simulink model "PMSM_18bMRASV20190225"  (R2020a)
settings: Solver=ode3  StartTime=0.0  StopTime=50  FixedStep=Ts  MaxStep=2e-5  MinStep=1e-5  RelTol=2e-3
InitFcn:
  | Ld=8.9e-3;
  | Lq=12.7e-3;
  | L=(Ld+Lq)/2;
  | poles=3;
  | R=0.85;
  | flux=0.1216;
  | Ts=1e-5;
model workspace (MAT data in the model file):
  Tl2 = [0 -0.0065 -0.013 -0.0195 -0.026 -0.0325 -0.039 -0.0455 -0.052 -0.0585 -0.065 -0.0715 ... (360 elements, 1x360)]
libraries: powerlib x19, powerlib_extras x16, simulink x8
settings Model: SimulationMode=accelerator  Creator=Paladin611  LastModifiedBy=Administrator
settings SolverCC: InitialStep=1e-5  MaxConsecutiveZCs=2000  ShapePreserveControl=EnableAll  AutoInsertRateTranBlk=on  InsertRTBMode=Always
settings DataIOCC: SaveFormat=Array  ReturnWorkspaceOutputs=off
settings OptimizationCC: DefaultParameterBehavior=Inlined  EnhancedBackFolding=on  PassReuseOutputArgsAs=Individual arguments  ExpressionDepthLimit=2147483647  ZeroExternalMemoryAtStartup=off  ZeroInternalMemoryAtStartup=off  InitFltsAndDblsToZero=on  EfficientMapNaN2IntZero=off  OptimizeBlockOrder=speed  DifferentSizesBufferReuse=on  OptimizationCustomize=off  EfficientTunableParamExpr=on
settings DebuggingCC: SaveWithParameterizedLinksMsg=none  UnderspecifiedInitializationDetection=Classic  MergeDetectMultiDrivingBlocksExec=none  SignalResolutionControl=TryResolveAllWithWarning  SolverPrmCheckMsg=warning  MultiTaskCondExecSysMsg=none  ParameterTunabilityLossMsg=error  FcnCallInpInsideContextMsg=warning  StateNameClashWarn=warning  SFUnexpectedBacktrackingDiag=warning  SFNoUnconditionalDefaultTransitionDiag=warning  SFExecutionAtInitializationDiag=none  ArithmeticOperatorsInVariantConditions=warning
settings HardwareCC: ProdBitPerPointer=32  ProdBitPerSizeT=32  ProdBitPerPtrDiffT=32  ProdLargestAtomicFloat=None  ProdIntDivRoundTo=Undefined  ProdEndianess=Unspecified  ProdWordSize=32  ProdHWDeviceType=32-bit Generic  TargetBitPerPointer=64  TargetBitPerSizeT=64  TargetBitPerPtrDiffT=64  TargetLongLongMode=on  TargetIntDivRoundTo=Zero  TargetEndianess=LittleEndian  TargetWordSize=64  TargetHWDeviceType=MATLAB Host  ProdEqTarget=off
settings ModelReferenceCC: PropagateSignalLabelsOutOfModel=off
settings SFSimCC: SimUseLocalCustomCode=off  MATLABDynamicMemAlloc=off  CustomCodeUndefinedFunction=UseInterfaceOnly
settings RTWCC: SystemTargetFile=ert.tlc  TemplateMakefile=ert_default_tmf  GenerateReport=on  RTWUseLocalCustomCode=off  IncludeHyperlinkInReport=on  LaunchReport=on  GenerateTraceInfo=on  GenerateTraceReport=on  GenerateTraceReportSl=on  GenerateTraceReportSf=on  GenerateTraceReportEml=on
settings CodeAppCC: ForceParamTrailComments=on  IgnoreCustomStorageClasses=off  MaxIdLength=128  OperatorAnnotations=on  SimulinkDataObjDesc=on  SFDataObjDesc=on  InsertBlockDesc=on
settings ERTTargetCC: GenerateSampleERTMain=on  InlinedParameterPlacement=NonHierarchical  ERTCustomFileTemplate=example_file_process.tlc
settings ConfigComp: CovMetricSettings=dw  CovHtmlReporting=on  CovSaveCumulativeToWorkspaceVar=on  CovSaveSingleToWorkspaceVar=on  CovExternalEMLEnable=off  CovSFcnEnable=off
settings SimscapeCC: SimscapeNormalizeSystem=off

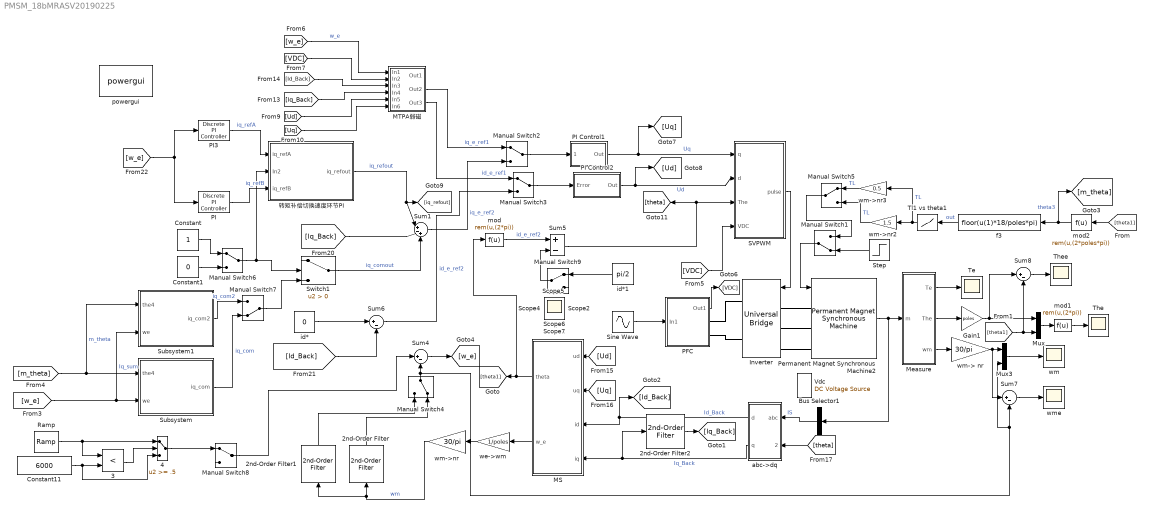
== system PMSM_18bMRASV20190225 ==
  "  3" : RelationalOperator  Operator=<  OutDataTypeStr=boolean  RndMeth=Nearest
  " Tl1 vs theta1" : Lookup  InputValues=0:359  Table=Tl2
  2nd-Order Filter : powerlib_extras/Control  Blocks/2nd-Order Filter  FilterType=Lowpass  Fo=30  Zeta=0.707  Initialize=off  Vac_Init=[1 45 60]  Vdc_Init=-0.5  PlotResponse=off  param1=[1 500 1]
      settings: SourceProductBaseCode=PS
  2nd-Order Filter1 : powerlib_extras/Control  Blocks/2nd-Order Filter  FilterType=Lowpass  Fo=800  Zeta=0.707  Initialize=off  Vac_Init=[1 45 60]  Vdc_Init=-0.5  PlotResponse=off  param1=[1 500 1]
      settings: SourceProductBaseCode=PS
  2nd-Order Filter2 : powerlib_extras/Control  Blocks/2nd-Order Filter  FilterType=Lowpass  Fo=800  Zeta=0.707  Initialize=off  Vac_Init=[1 45 60]  Vdc_Init=-0.5  PlotResponse=off  param1=[1 500 1]
      settings: SourceProductBaseCode=PS
  4 : Switch  Threshold=.5
  Bus Selector1 : BusSelector  OutputSignals=Stator current is_a (A),Stator current is_b (A),Stator current is_c (A)  OutputAsBus=on
  Constant : Constant
  Constant1 : Constant  Value=0
  Constant11 : Constant  Value=6000
  Gain1 : Gain  Gain=poles
  Inverter : powerlib/Power Electronics/Universal Bridge  Arms=3  SnubberResistance=1e5  SnubberCapacitance=inf  Device=IGBT / Diodes  Ron=1e-3  Lon=0  ForwardVoltages="[  0  0  ]"  ForwardVoltage=0  GTOparameters=[ 10e-6 , 20e-6 ]  IGBTparameters=[ 1e-6 , 2e-6 ]  Measurements=None  Measurements_2=None  converterType=Rectifier
  MS : Subsystem
  MTPA弱磁 : Subsystem
  Manual Switch1 : ManualSwitch  CurrentSetting=0
  Manual Switch{2..3,5..6,8..9} (6 alike) : ManualSwitch
  Manual Switch4 : ManualSwitch  CurrentSetting=0
  Manual Switch7 : ManualSwitch  CurrentSetting=0
  Measure : Subsystem
  Mux : Mux  Inputs=2
  Mux3 : Mux  Inputs=2
  PFC : Subsystem
  PI : powerlib_extras/Discrete  Control Blocks/Discrete PI Controller  Kp=0.002  Ki=0.0002  Par_Limits=[200 -200]  Init=0  Ts=Ts
  PI Control1 : Subsystem  mask(PI Control){Kp=Lq*2000, Ki=R*2000, Kc=3, UpperLimit=400, LowerLimit=-400}
      mask prompts: Kp "PI_Kp:"; Ki "PI_Ki:"; Kc "PI_Kc:"; UpperLimit "MAX:"; LowerLimit "MIN:"
      mask help:
      | PI Control
      |
      | CopyRight:maxthonzwq 2012/03/22
  PI Control2 : Subsystem  mask(PI Control){Kp=Ld*2000, Ki=R*2000, Kc=3, UpperLimit=400, LowerLimit=-400}
      mask prompts: Kp "PI_Kp:"; Ki "PI_Ki:"; Kc "PI_Kc:"; UpperLimit "MAX:"; LowerLimit "MIN:"
      mask help:
      | PI Control
      |
      | CopyRight:maxthonzwq 2012/03/22
  PI3 : powerlib_extras/Discrete  Control Blocks/Discrete PI Controller  Kp=0.03  Ki=0.002  Par_Limits=[200 -200]  Init=0  Ts=Ts
  Permanent Magnet Synchronous Machine2 : powerlib/Machines/Permanent Magnet Synchronous Machine  NbPhases=3  FluxDistribution=Sinusoidal  RotorType=Salient-pole  MechanicalLoad=Torque Tm  PresetModel=No  ShowDetailedParameters=on  MeasurementBus=off  Resistance=R  Inductance=8.5e-3  dqInductances=[Ld Lq]  La=0.00085  MachineConstant=Flux linkage established by magnets (V.s)  Flux=0.175  VoltageCst=126.966  TorqueCst=1.05  Flat=120  Mechanical=[3.4e-4,0,poles,0]  PolePairs=4  InitialConditions=[0,0, 0,0]  InitialConditions5ph=[0 0 0 0 0 0]  RefAngle=Aligned with phase A axis (original Park)  IterativeDiscreteModel=Trapezoidal non iterative  TsBlock=-1  TsPowergui=0
  Ramp : simulink/Sources/Ramp  slope=1000  start=0  InitialOutput=1
  SVPWM : Subsystem
  Sine Wave : Sin  Frequency=50*2*pi  SampleTime=0
  Step : Step  Time=0  Before=0.3  SampleTime=0
  Subsystem : Subsystem
  Subsystem1 : Subsystem
  Sum1 : Sum  Inputs=|+-+
  Sum{4,6..8} (4 alike) : Sum  Inputs=|+-
  Sum5 : Sum  Inputs=+-
  Switch1 : Switch  Criteria=u2 > Threshold
  Te : Scope
  The : Scope
  Thee : Scope
  Vdc : powerlib/Electrical Sources/DC Voltage Source  Amplitude=311  Measurements=None
  abc->dq : Subsystem
  f3 : Fcn  Expr=floor(u(1)*18/poles*pi)  SampleTime=0.0001
  id* : Constant  Value=0
  id*1 : Constant  Value=pi/2
  mod : Fcn  Expr=rem(u,(2*pi))
  mod1 : Fcn  Expr=rem(u,(2*pi))
  mod2 : Fcn  Expr=rem(u,(2*poles*pi))
  powergui : powerlib/powergui  Priority=1  SimulationMode=Discrete  SampleTime=Ts  frequency=60  Iterations=50  frequencyindice=0  Pbase=100e6  ErrMax=1e-4  UnitsV=kV  UnitsW=MW  buscounter=0  FunctionMessages=off  echomessages=off  EnableUseOfTLC=off  CurrentSourceSwitches=on  DisableSnubberDevices=off  DisableRonSwitches=off  DisableVfSwitches=off  DisplayEquations=off  AutomaticDiscreteSolvers=off  SolverType=Tustin  Interpol=off  ExternalGateDelay=off  methode=off  Ts=0  x0status=blocks  SPID=off  SwTol=0  HookPort=off  NonlinearTolerance=1e-4  nMaxIteration=100  ContinueOnMaxIteration=off  RestoreLinks=warning  ResistiveCurrentMeasurement=off  Frange=[0:2:500]  Ylog=off  Xlog=on  ShowGrid=off  save=off  variable=ZData  structure=0  ZoomFFT=off  StartTime=0.0  cycles=1  DisplayStyle=1  fundamental=60  FreqAxis=off  MaxFrequency=1000  frequencyindicesteady=1  RmsSteady=1  display=off
  we->wm : Gain  Gain=1/poles
  wm : Scope
  wm-> nr : Gain  Gain=30/pi
  wm->nr : Gain  Gain=30/pi
  wm->nr2 : Gain  Gain=1.5
  wm->nr3 : Gain  Gain=0.5
  wme : Scope
  转矩补偿切换速度环节PI : Subsystem
  Scope{,1..2,4..7} (7 alike) : Scope
  wires:
  Permanent Magnet Synchronous Machine2/1 -> Measure/1(m), Bus Selector1/1
  id*/1 -> Sum6/1
  SVPWM/1(pulse) -> Inverter/1
  abc->dq/2(q) -> 2nd-Order Filter2/1, MS/4(iq)  "Iq_Back"
  MS/2(w_e) -> we->wm/1
  we->wm/1 -> wm->nr/1
  PI Control1/1(Out) -> SVPWM/1(q), [Uq]  "Uq"
  PI Control2/1(Out) -> [Ud], SVPWM/2(d)  "Ud"
  Measure/1(Te) -> Te/1
  Measure/2(The) -> Gain1/1
  Bus Selector1/1 -> abc->dq/1(abc)  "IS"
  Measure/3(wm) -> wm-> nr/1
  f3/1 -> " Tl1 vs theta1"/1  "out"
  [theta1] -> mod2/1
  Switch1/1 -> Sum1/3  "iq_comout"
  mod2/1 -> [m_theta], f3/1  "theta3"
  Step/1 -> Manual Switch1/2
  " Tl1 vs theta1"/1 -> wm->nr2/1, wm->nr3/1  "TL"
  PI3/1 -> 转矩补偿切换速度环节PI/1(iq_refA)  "iq_refA"
  Manual Switch6/1 -> 转矩补偿切换速度环节PI/2(In2), Switch1/2
  PI/1 -> 转矩补偿切换速度环节PI/3(iq_refB)  "iq_refB"
  转矩补偿切换速度环节PI/1(iq_refout) -> [iq_refout], Sum1/1  "iq_refout"
  [VDC] -> SVPWM/4(VDC)
  [Ud] -> MS/1(ud)
  [Uq] -> MS/2(uq)
  [theta] -> abc->dq/2(theta)
  [Id_Back] -> Sum6/2
  [Iq_Back] -> Sum1/2
  [w_e] -> PI/1, PI3/1
  Sine Wave/1 -> PFC/1(In1)
  Sum1/1 -> Manual Switch2/2  "iq_e_ref2"
  Manual Switch3/1 -> PI Control2/1(Error)
  Sum6/1 -> Manual Switch3/2  "id_e_ref2"
  [VDC] -> MTPA弱磁/2(In2)
  MTPA弱磁/2(Out2) -> Manual Switch2/1  "iq_e_ref1"
  MTPA弱磁/3(Out3) -> Manual Switch3/1  "id_e_ref1"
  [Id_Back] -> MTPA弱磁/3(In3)
  [Iq_Back] -> MTPA弱磁/4(In4)
  [Ud] -> MTPA弱磁/5(In5)
  [Uq] -> MTPA弱磁/6(In6)
  PFC/1(Out1) -> [VDC]
  abc->dq/1(d) -> MS/3(id), [Id_Back]  "Id_Back"
  Sum4/1 -> [w_e]
  [w_e] -> MTPA弱磁/1(In1)  "w_e"
  2nd-Order Filter/1 -> Manual Switch4/2
  wm->nr/1 -> 2nd-Order Filter1/1, 2nd-Order Filter/1  "wm"
  [m_theta] -> Subsystem/1(the4), Subsystem1/1(the4)  "m_theta"
  [w_e] -> Subsystem/2(we), Subsystem1/2(we)  "Iq_sum"
  Manual Switch1/1 -> Permanent Magnet Synchronous Machine2/1
  Manual Switch5/1 -> Manual Switch1/1
  wm->nr2/1 -> Manual Switch5/2  "TL"
  wm->nr3/1 -> Manual Switch5/1  "TL"
  Constant/1 -> Manual Switch6/1
  Constant1/1 -> Manual Switch6/2
  Subsystem1/1(iq_com2) -> Manual Switch7/1  "iq_com2"
  Subsystem/1(iq_com) -> Manual Switch7/2  "iq_com"
  Manual Switch7/1 -> Switch1/3
  2nd-Order Filter1/1 -> Manual Switch4/1
  2nd-Order Filter2/1 -> [Iq_Back]
  4/1 -> Manual Switch8/1
  Ramp/1 -> "  3"/1, 4/1
  Constant11/1 -> "  3"/2, 4/3
  "  3"/1 -> 4/2
  Manual Switch8/1 -> Sum4/1
  Manual Switch2/1 -> PI Control1/1(Error)
  Mux3/1 -> wm/1
  Sum7/1 -> wme/1
  Manual Switch4/1 -> Mux3/2, Sum7/2, Sum4/2
  Sum8/1 -> Thee/1
  wm-> nr/1 -> Sum7/1, Mux3/1
  mod1/1 -> The/1
  Mux/1 -> mod1/1
  MS/1(theta) -> mod/1, [theta1]
  Gain1/1 -> Mux/1, Sum8/1
  mod/1 -> Sum5/1  "id_e_ref2"
  Sum5/1 -> SVPWM/3(The), [theta]
  Manual Switch9/1 -> Sum5/2
  id*1/1 -> Manual Switch9/1
  [theta1] -> Sum8/2, Mux/2
  connections:
  Permanent Magnet Synchronous Machine2/LConn1 -- Inverter/LConn1
  Permanent Magnet Synchronous Machine2/LConn2 -- Inverter/LConn2
  Permanent Magnet Synchronous Machine2/LConn3 -- Inverter/LConn3
  Inverter/RConn1 -- PFC/RConn1
  Inverter/RConn2 -- PFC/RConn2

== system PMSM_18bMRASV20190225/MS ==
  ud : Inport
  uq : Inport  Port=2
  id : Inport  Port=3
  iq : Inport  Port=4
  Integrator : Integrator
  MRAS : Subsystem
  Manual Switch1 : ManualSwitch  CurrentSetting=0
  we : Subsystem
  we1 : Subsystem
  theta : Outport  VectorParamsAs1DForOutWhenUnconnected=off
  w_e : Outport  Port=2  VectorParamsAs1DForOutWhenUnconnected=off
  wires:
  ud/1 -> MRAS/1(ud)
  iq/1 -> we/2(iq), we1/2(iq)
  uq/1 -> MRAS/2(uq)
  Integrator/1 -> theta/1
  MRAS/2(i_q) -> we/4(i_q), we1/4(i_q)
  MRAS/1(i_d) -> we/3(i_d), we1/3(i_d)
  id/1 -> we/1(id), we1/1(id)
  Manual Switch1/1 -> MRAS/3(we), w_e/1, Integrator/1
  we/1(w_e) -> Manual Switch1/2
  we1/1(w_e) -> Manual Switch1/1

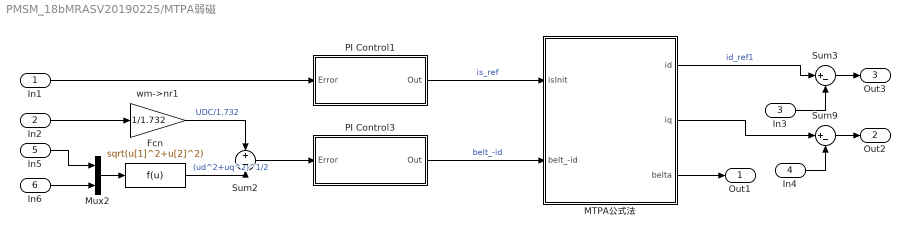
== system PMSM_18bMRASV20190225/MTPA弱磁 ==
  In1 : Inport
  In2 : Inport  Port=2
  In3 : Inport  Port=3
  In4 : Inport  Port=4
  In5 : Inport  Port=5
  In6 : Inport  Port=6
  Fcn : Fcn  Expr=sqrt(u[1]^2+u[2]^2)
  MTPA公式法 : Subsystem
  Mux2 : Mux  Inputs=2
  PI Control1 : Subsystem  mask(PI Control){Kp=0.05, Ki=0.004, Kc=3, UpperLimit=200, LowerLimit=-200}
      mask prompts: Kp "PI_Kp:"; Ki "PI_Ki:"; Kc "PI_Kc:"; UpperLimit "MAX:"; LowerLimit "MIN:"
      mask help:
      | PI Control
      |
      | CopyRight:maxthonzwq 2012/03/22
  PI Control3 : Subsystem  mask(PI Control){Kp=0.05, Ki=0.002, Kc=3, UpperLimit=200, LowerLimit=-200}
      mask prompts: Kp "PI_Kp:"; Ki "PI_Ki:"; Kc "PI_Kc:"; UpperLimit "MAX:"; LowerLimit "MIN:"
      mask help:
      | PI Control
      |
      | CopyRight:maxthonzwq 2012/03/22
  Sum2 : Sum  Inputs=+-
  Sum3 : Sum  Inputs=|+-
  Sum9 : Sum  Inputs=|+-
  wm->nr1 : Gain  Gain=1/1.732
  Out1 : Outport  VectorParamsAs1DForOutWhenUnconnected=off
  Out2 : Outport  Port=2  VectorParamsAs1DForOutWhenUnconnected=off
  Out3 : Outport  Port=3  VectorParamsAs1DForOutWhenUnconnected=off
  wires:
  wm->nr1/1 -> Sum2/1  "UDC/1.732"
  Fcn/1 -> Sum2/2  "(ud^2+uq^2)^1/2"
  PI Control3/1(Out) -> MTPA公式法/2(belt_-id)  "belt_-id"
  Sum2/1 -> PI Control3/1(Error)
  MTPA公式法/3(belta) -> Out1/1
  Sum3/1 -> Out3/1
  MTPA公式法/2(iq) -> Sum9/1
  Mux2/1 -> Fcn/1
  MTPA公式法/1(id) -> Sum3/1  "id_ref1"
  In3/1 -> Sum3/2
  Sum9/1 -> Out2/1
  In5/1 -> Mux2/1
  In2/1 -> wm->nr1/1
  In4/1 -> Sum9/2
  In1/1 -> PI Control1/1(Error)
  In6/1 -> Mux2/2
  PI Control1/1(Out) -> MTPA公式法/1(isInit)  "is_ref"

== system PMSM_18bMRASV20190225/Measure ==
  m : Inport
  Bus Selector : BusSelector  OutputSignals=Electromagnetic torque Te (N*m),Rotor angle thetam (rad),Rotor speed wm (rad/s)
  Te : Outport  VectorParamsAs1DForOutWhenUnconnected=off
  The : Outport  Port=2  VectorParamsAs1DForOutWhenUnconnected=off
  wm : Outport  Port=3  VectorParamsAs1DForOutWhenUnconnected=off
  wires:
  Bus Selector/1 -> Te/1  "<Electromagnetic torque Te (N*m)>"
  Bus Selector/3 -> wm/1  "<Rotor speed wm (rad/s)>"
  Bus Selector/2 -> The/1  "<Rotor angle thetam (rad)>"
  m/1 -> Bus Selector/1

== system PMSM_18bMRASV20190225/PFC ==
  In1 : Inport
  2nd-Order Filter : powerlib_extras/Control  Blocks/2nd-Order Filter  FilterType=Lowpass  Fo=20  Zeta=0.707  Initialize=off  Vac_Init=[1 45 60]  Vdc_Init=-0.5  PlotResponse=off  param1=[1 500 1]
      settings: SourceProductBaseCode=PS
  Constant : Constant  Value=350
  PFC : Subsystem
  Sum11 : Sum  Inputs=|-+
  Voltage Measurement1 : powerlib/Measurements/Voltage Measurement  PhasorSimulation=off  OutputType=Complex  PSBequivalent=0
  Conn1 : PMIOPort  Side=Right
  Conn2 : PMIOPort  Port=2  Side=Right
  Out1 : Outport  VectorParamsAs1DForOutWhenUnconnected=off
  wires:
  Sum11/1 -> PFC/2(In2)
  Constant/1 -> Sum11/2
  2nd-Order Filter/1 -> PFC/3(VDC), Sum11/1  "VDC"
  In1/1 -> PFC/1(In1)
  Voltage Measurement1/1 -> Out1/1, 2nd-Order Filter/1  "VDC1"
  connections:
  Voltage Measurement1/LConn2 -- Conn2/RConn1 -- PFC/RConn2
  Voltage Measurement1/LConn1 -- Conn1/RConn1 -- PFC/RConn1

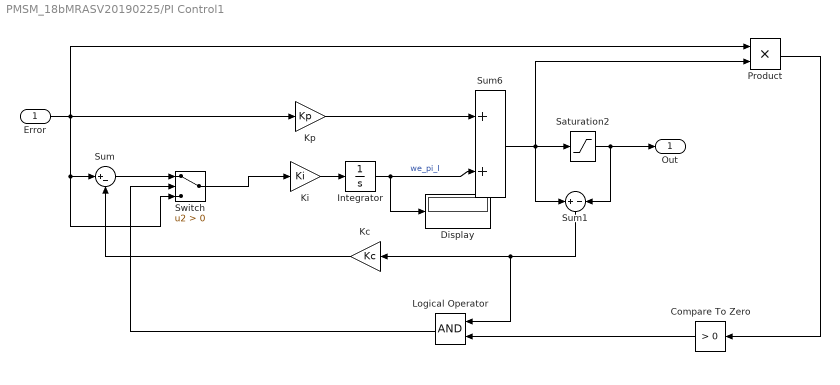
== system PMSM_18bMRASV20190225/PI Control1 ==
  Error : Inport
  Compare To Zero : simulink/Logic and Bit Operations/Compare To Zero  relop=>  OutDataTypeStr=uint8  ZeroCross=off
  Display : Display
  Integrator : Integrator
  Kc : Gain  Gain=Kc  OutDataTypeStr=Inherit: Same as input  ParamDataTypeStr=Inherit: Same as input
  Ki : Gain  Gain=Ki  OutDataTypeStr=Inherit: Same as input  ParamDataTypeStr=Inherit: Same as input
  Kp : Gain  Gain=Kp  OutDataTypeStr=Inherit: Same as input  ParamDataTypeStr=Inherit: Same as input
  Logical Operator : Logic  AllPortsSameDT=off  OutDataTypeStr=boolean
  Product : Product  RndMeth=Zero
  Saturation2 : Saturate  UpperLimit=UpperLimit  LowerLimit=LowerLimit
  Sum : Sum  Inputs=|+-  OutDataTypeStr=Inherit: Same as first input
  Sum1 : Sum  Inputs=+-  OutDataTypeStr=Inherit: Same as first input
  Sum6 : Sum  InputSameDT=on  SaturateOnIntegerOverflow=on  OutDataTypeStr=Inherit: Same as first input
  Switch : Switch  Criteria=u2 > Threshold
  Out : Outport
  wires:
  Compare To Zero/1 -> Logical Operator/2
  Product/1 -> Compare To Zero/1
  Kc/1 -> Sum/2
  Ki/1 -> Integrator/1
  Saturation2/1 -> Out/1, Sum1/2
  Kp/1 -> Sum6/1
  Sum6/1 -> Product/2, Sum1/1, Saturation2/1
  Integrator/1 -> Sum6/2, Display/1  "we_pi_I"
  Sum1/1 -> Kc/1, Logical Operator/1
  Error/1 -> Kp/1, Product/1, Sum/1, Switch/3
  Logical Operator/1 -> Switch/2
  Sum/1 -> Switch/1
  Switch/1 -> Ki/1

== system PMSM_18bMRASV20190225/PI Control2 ==
  Error : Inport
  Compare To Zero : simulink/Logic and Bit Operations/Compare To Zero  relop=>  OutDataTypeStr=uint8  ZeroCross=off
  Display : Display
  Integrator : Integrator
  Kc : Gain  Gain=Kc  OutDataTypeStr=Inherit: Same as input  ParamDataTypeStr=Inherit: Same as input
  Ki : Gain  Gain=Ki  OutDataTypeStr=Inherit: Same as input  ParamDataTypeStr=Inherit: Same as input
  Kp : Gain  Gain=Kp  OutDataTypeStr=Inherit: Same as input  ParamDataTypeStr=Inherit: Same as input
  Logical Operator : Logic  AllPortsSameDT=off  OutDataTypeStr=boolean
  Product : Product  RndMeth=Zero
  Saturation2 : Saturate  UpperLimit=UpperLimit  LowerLimit=LowerLimit
  Sum : Sum  Inputs=|+-  OutDataTypeStr=Inherit: Same as first input
  Sum1 : Sum  Inputs=+-  OutDataTypeStr=Inherit: Same as first input
  Sum6 : Sum  InputSameDT=on  SaturateOnIntegerOverflow=on  OutDataTypeStr=Inherit: Same as first input
  Switch : Switch  Criteria=u2 > Threshold
  Out : Outport
  wires:
  Compare To Zero/1 -> Logical Operator/2
  Product/1 -> Compare To Zero/1
  Kc/1 -> Sum/2
  Ki/1 -> Integrator/1
  Saturation2/1 -> Out/1, Sum1/2
  Kp/1 -> Sum6/1
  Sum6/1 -> Product/2, Sum1/1, Saturation2/1
  Integrator/1 -> Sum6/2, Display/1  "we_pi_I"
  Sum1/1 -> Kc/1, Logical Operator/1
  Error/1 -> Kp/1, Product/1, Sum/1, Switch/3
  Logical Operator/1 -> Switch/2
  Sum/1 -> Switch/1
  Switch/1 -> Ki/1

== system PMSM_18bMRASV20190225/SVPWM ==
  q : Inport
  d : Inport  Port=2
  The : Inport  Port=3
  VDC : Inport  Port=4
  Fcn : Fcn  Expr=cos(u[3])*u[2]-sin(u[3])*u[1]
  Fcn1 : Fcn  Expr=cos(u[3])*u[1]+sin(u[3])*u[2]
  Mux1 : Mux  Inputs=3
  SVPWM : Subsystem  Tag=SVPWM  mask{F=6, Vdc=350}
      mask prompts: F "Chopping　Frequency(KHz)"; Vdc "DC Voltage(V)"
  pulse : Outport  VectorParamsAs1DForOutWhenUnconnected=off
  wires:
  The/1 -> Mux1/3
  Mux1/1 -> Fcn1/1, Fcn/1
  d/1 -> Mux1/2
  q/1 -> Mux1/1
  Fcn/1 -> SVPWM/1(Ualfa)
  Fcn1/1 -> SVPWM/2(Ubeta)
  SVPWM/1(pulse) -> pulse/1
  VDC/1 -> SVPWM/3(VDC)

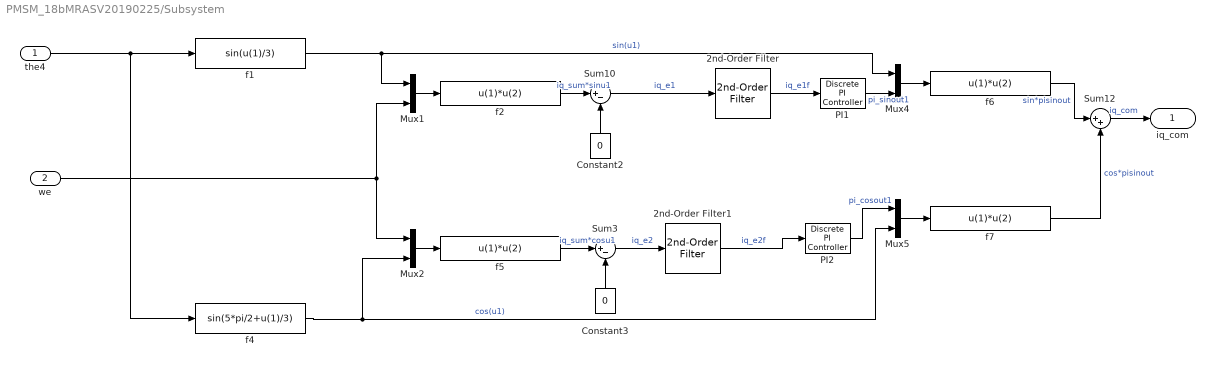
== system PMSM_18bMRASV20190225/Subsystem ==
  the4 : Inport
  we : Inport  Port=2
  2nd-Order Filter : powerlib_extras/Control  Blocks/2nd-Order Filter  FilterType=Lowpass  Fo=800  Zeta=0.707  Initialize=off  Vac_Init=[1 45 60]  Vdc_Init=-0.5  PlotResponse=off  param1=[1 500 1]
      settings: SourceProductBaseCode=PS
  2nd-Order Filter1 : powerlib_extras/Control  Blocks/2nd-Order Filter  FilterType=Lowpass  Fo=800  Zeta=0.707  Initialize=off  Vac_Init=[1 45 60]  Vdc_Init=-0.5  PlotResponse=off  param1=[1 500 1]
      settings: SourceProductBaseCode=PS
  Constant2 : Constant  Value=0
  Constant3 : Constant  Value=0
  Mux{1..2,4..5} (4 alike) : Mux  Inputs=2
  PI1 : powerlib_extras/Discrete  Control Blocks/Discrete PI Controller  Kp=0.03  Ki=0.001  Par_Limits=[200 -200]  Init=0  Ts=Ts
  PI2 : powerlib_extras/Discrete  Control Blocks/Discrete PI Controller  Kp=0.03  Ki=0.001  Par_Limits=[100 -100]  Init=0  Ts=Ts
  Sum10 : Sum  Inputs=|+-
  Sum12 : Sum  Inputs=|++
  Sum3 : Sum  Inputs=|+-
  f1 : Fcn  Expr=sin(u(1)/3)  SampleTime=0.0001
  f{2,5..7} (4 alike) : Fcn  Expr=u(1)*u(2)  SampleTime=0.0001
  f4 : Fcn  Expr=sin(5*pi/2+u(1)/3)  SampleTime=0.0001
  iq_com : Outport
  wires:
  Constant3/1 -> Sum3/2
  f4/1 -> Mux5/2, Mux2/2  "cos(u1)"
  f2/1 -> Sum10/1  "iq_sum*sinu1"
  Sum3/1 -> 2nd-Order Filter1/1  "iq_e2"
  we/1 -> Mux2/1, Mux1/2
  Constant2/1 -> Sum10/2
  f5/1 -> Sum3/1  "iq_sum*cosu1"
  f6/1 -> Sum12/1  "sin*pisinout"
  PI1/1 -> Mux4/2  "pi_sinout1"
  f7/1 -> Sum12/2  "cos*pisinout"
  PI2/1 -> Mux5/1  "pi_cosout1"
  Mux5/1 -> f7/1
  Mux1/1 -> f2/1
  Mux4/1 -> f6/1
  f1/1 -> Mux1/1, Mux4/1  "sin(u1)"
  2nd-Order Filter1/1 -> PI2/1  "iq_e2f"
  Mux2/1 -> f5/1
  Sum12/1 -> iq_com/1  "iq_com"
  2nd-Order Filter/1 -> PI1/1  "iq_e1f"
  Sum10/1 -> 2nd-Order Filter/1  "iq_e1"
  the4/1 -> f4/1, f1/1

== system PMSM_18bMRASV20190225/Subsystem1 ==
  the4 : Inport
  we : Inport  Port=2
  2nd-Order Filter : powerlib_extras/Control  Blocks/2nd-Order Filter  FilterType=Lowpass  Fo=800  Zeta=0.707  Initialize=off  Vac_Init=[1 45 60]  Vdc_Init=-0.5  PlotResponse=off  param1=[1 500 1]
      settings: SourceProductBaseCode=PS
  Constant2 : Constant  Value=0
  Mux1 : Mux  Inputs=2
  PI1 : powerlib_extras/Discrete  Control Blocks/Discrete PI Controller  Kp=0.03  Ki=0.003  Par_Limits=[200 -200]  Init=0  Ts=Ts
  Sum10 : Sum  Inputs=|+-
  f1 : Fcn  Expr=sin(u(1)/6)  SampleTime=0.0001
  f2 : Fcn  Expr=u(1)*u(2)  SampleTime=0.0001
  iq_com2 : Outport
  wires:
  we/1 -> Mux1/2
  Constant2/1 -> Sum10/2
  Mux1/1 -> f2/1
  2nd-Order Filter/1 -> PI1/1  "iq_e2f"
  Sum10/1 -> 2nd-Order Filter/1
  the4/1 -> f1/1
  f1/1 -> Mux1/1  "sin(u1)"
  f2/1 -> Sum10/1  "we*abs(sin)"
  PI1/1 -> iq_com2/1  "we*abs(sin)"

== system PMSM_18bMRASV20190225/abc->dq ==
  abc : Inport
  theta : Inport  Port=2
  Fcn : Fcn  Expr=2/3*(u[1]*cos(u[4])+u[2]*cos(u[4]-2*pi/3)+u[3]*cos(u[4]+2*pi/3))
  Fcn1 : Fcn  Expr=2/3*(-u[1]*sin(u[4])-u[2]*sin(u[4]-2*pi/3)-u[3]*sin(u[4]+2*pi/3))
  Mux3 : Mux  Inputs=2
  d : Outport  VectorParamsAs1DForOutWhenUnconnected=off
  q : Outport  Port=2  VectorParamsAs1DForOutWhenUnconnected=off
  wires:
  Mux3/1 -> Fcn1/1, Fcn/1
  theta/1 -> Mux3/2
  Fcn/1 -> d/1
  Fcn1/1 -> q/1
  abc/1 -> Mux3/1

== system PMSM_18bMRASV20190225/转矩补偿切换速度环节PI ==
  iq_refA : Inport
  In2 : Inport  Port=2
  iq_refB : Inport  Port=3
  2nd-Order Filter : powerlib_extras/Control  Blocks/2nd-Order Filter  FilterType=Lowpass  Fo=800  Zeta=0.707  Initialize=off  Vac_Init=[1 45 60]  Vdc_Init=-0.5  PlotResponse=off  param1=[1 500 1]
      settings: SourceProductBaseCode=PS
  2nd-Order Filter1 : powerlib_extras/Control  Blocks/2nd-Order Filter  FilterType=Lowpass  Fo=800  Zeta=0.707  Initialize=off  Vac_Init=[1 45 60]  Vdc_Init=-0.5  PlotResponse=off  param1=[1 500 1]
      settings: SourceProductBaseCode=PS
  Switch2 : Switch  Criteria=u2 > Threshold
  iq_refout : Outport
  wires:
  Switch2/1 -> iq_refout/1
  2nd-Order Filter/1 -> Switch2/1  "iq_refA1"
  2nd-Order Filter1/1 -> Switch2/3  "iq_refB1"
  In2/1 -> Switch2/2
  iq_refA/1 -> 2nd-Order Filter/1
  iq_refB/1 -> 2nd-Order Filter1/1

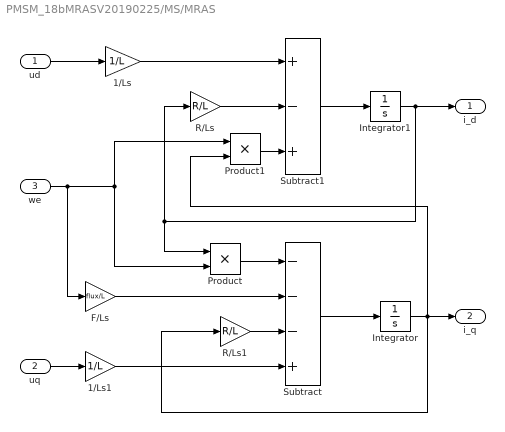
== system PMSM_18bMRASV20190225/MS/MRAS ==
  ud : Inport
  uq : Inport  Port=2
  we : Inport  Port=3
  1/Ls : Gain  Gain=1/L
  1/Ls1 : Gain  Gain=1/L
  F/Ls : Gain  Gain=flux/L
  Integrator : Integrator
  Integrator1 : Integrator
  Product : Product  RndMeth=Zero
  Product1 : Product  RndMeth=Zero
  R/Ls : Gain  Gain=R/L
  R/Ls1 : Gain  Gain=R/L
  Subtract : Sum  Inputs=---+
  Subtract1 : Sum  Inputs=+-+
  i_d : Outport  VectorParamsAs1DForOutWhenUnconnected=off
  i_q : Outport  Port=2  VectorParamsAs1DForOutWhenUnconnected=off
  wires:
  1/Ls1/1 -> Subtract/4
  Subtract/1 -> Integrator/1
  Subtract1/1 -> Integrator1/1
  1/Ls/1 -> Subtract1/1
  Product1/1 -> Subtract1/3
  R/Ls/1 -> Subtract1/2
  Product/1 -> Subtract/1
  R/Ls1/1 -> Subtract/3
  uq/1 -> 1/Ls1/1
  we/1 -> F/Ls/1, Product/2, Product1/1
  F/Ls/1 -> Subtract/2
  Integrator1/1 -> R/Ls/1, Product/1, i_d/1
  ud/1 -> 1/Ls/1
  Integrator/1 -> R/Ls1/1, i_q/1, Product1/2

== system PMSM_18bMRASV20190225/MS/we ==
  id : Inport
  iq : Inport  Port=2
  i_d : Inport  Port=3
  i_q : Inport  Port=4
  F/Ls : Gain  Gain=flux/L
  Integrator : Integrator
  Ki : Gain  Gain=0.5
  Kp : Gain  Gain=0.3
  Product2 : Product  RndMeth=Zero
  Product3 : Product  RndMeth=Zero
  Subtract1 : Sum  Inputs=+--
  Subtract2 : Sum
  Subtract3 : Sum  Inputs=+-
  w_e : Outport  VectorParamsAs1DForOutWhenUnconnected=off
  wires:
  id/1 -> Product2/1
  i_q/1 -> Subtract3/2, Product2/2
  iq/1 -> Subtract3/1, Product3/1
  i_d/1 -> Product3/2
  Subtract3/1 -> F/Ls/1
  F/Ls/1 -> Subtract1/3
  Subtract1/1 -> Ki/1, Kp/1
  Ki/1 -> Integrator/1
  Integrator/1 -> Subtract2/1
  Kp/1 -> Subtract2/2
  Product2/1 -> Subtract1/1
  Product3/1 -> Subtract1/2
  Subtract2/1 -> w_e/1

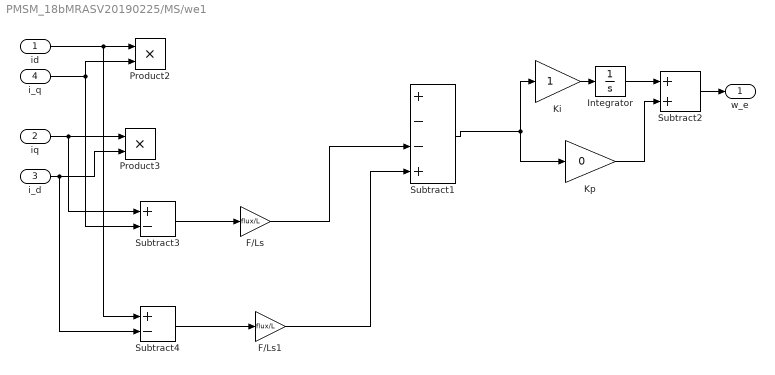
== system PMSM_18bMRASV20190225/MS/we1 ==
  id : Inport
  iq : Inport  Port=2
  i_d : Inport  Port=3
  i_q : Inport  Port=4
  F/Ls : Gain  Gain=flux/L
  F/Ls1 : Gain  Gain=flux/L
  Integrator : Integrator
  Ki : Gain
  Kp : Gain  Gain=0
  Product2 : Product  RndMeth=Zero
  Product3 : Product  RndMeth=Zero
  Subtract1 : Sum  Inputs=+--+
  Subtract2 : Sum
  Subtract3 : Sum  Inputs=+-
  Subtract4 : Sum  Inputs=+-
  w_e : Outport  VectorParamsAs1DForOutWhenUnconnected=off
  wires:
  id/1 -> Subtract4/1, Product2/1
  i_q/1 -> Subtract3/2, Product2/2
  iq/1 -> Subtract3/1, Product3/1
  i_d/1 -> Subtract4/2, Product3/2
  Subtract3/1 -> F/Ls/1
  F/Ls/1 -> Subtract1/3
  Subtract1/1 -> Kp/1, Ki/1
  Ki/1 -> Integrator/1
  Integrator/1 -> Subtract2/1
  Kp/1 -> Subtract2/2
  Subtract2/1 -> w_e/1
  Subtract4/1 -> F/Ls1/1
  F/Ls1/1 -> Subtract1/4

== system PMSM_18bMRASV20190225/MTPA弱磁/MTPA公式法 ==
  isInit : Inport
  belt_-id : Inport  Port=2
  MTPA : Subsystem
  Subsystem1 : Subsystem
  Sum5 : Sum  Inputs=+-
  id : Outport
  iq : Outport  Port=2
  belta : Outport  Port=3
  wires:
  MTPA/1(belta) -> Sum5/1  "beltref"
  isInit/1 -> MTPA/1(is), Subsystem1/2(is)
  belt_-id/1 -> Sum5/2
  Subsystem1/1(id) -> id/1
  Subsystem1/2(iq) -> iq/1
  Sum5/1 -> Subsystem1/1("belta "), belta/1  "beltout"

== system PMSM_18bMRASV20190225/MTPA弱磁/PI Control1 ==
  Error : Inport
  Compare To Zero : simulink/Logic and Bit Operations/Compare To Zero  relop=>  OutDataTypeStr=uint8  ZeroCross=off
  Display : Display
  Integrator : Integrator
  Kc : Gain  Gain=Kc  OutDataTypeStr=Inherit: Same as input  ParamDataTypeStr=Inherit: Same as input
  Ki : Gain  Gain=Ki  OutDataTypeStr=Inherit: Same as input  ParamDataTypeStr=Inherit: Same as input
  Kp : Gain  Gain=Kp  OutDataTypeStr=Inherit: Same as input  ParamDataTypeStr=Inherit: Same as input
  Logical Operator : Logic  AllPortsSameDT=off  OutDataTypeStr=boolean
  Product : Product  RndMeth=Zero
  Saturation2 : Saturate  UpperLimit=UpperLimit  LowerLimit=LowerLimit
  Sum : Sum  Inputs=|+-  OutDataTypeStr=Inherit: Same as first input
  Sum1 : Sum  Inputs=+-  OutDataTypeStr=Inherit: Same as first input
  Sum6 : Sum  InputSameDT=on  SaturateOnIntegerOverflow=on  OutDataTypeStr=Inherit: Same as first input
  Switch : Switch  Criteria=u2 > Threshold
  Out : Outport
  wires:
  Compare To Zero/1 -> Logical Operator/2
  Product/1 -> Compare To Zero/1
  Kc/1 -> Sum/2
  Ki/1 -> Integrator/1
  Saturation2/1 -> Out/1, Sum1/2
  Kp/1 -> Sum6/1
  Sum6/1 -> Product/2, Sum1/1, Saturation2/1
  Integrator/1 -> Sum6/2, Display/1  "we_pi_I"
  Sum1/1 -> Kc/1, Logical Operator/1
  Error/1 -> Kp/1, Product/1, Sum/1, Switch/3
  Logical Operator/1 -> Switch/2
  Sum/1 -> Switch/1
  Switch/1 -> Ki/1

== system PMSM_18bMRASV20190225/MTPA弱磁/PI Control3 ==
  Error : Inport
  Compare To Zero : simulink/Logic and Bit Operations/Compare To Zero  relop=>  OutDataTypeStr=uint8  ZeroCross=off
  Display : Display
  Integrator : Integrator
  Kc : Gain  Gain=Kc  OutDataTypeStr=Inherit: Same as input  ParamDataTypeStr=Inherit: Same as input
  Ki : Gain  Gain=Ki  OutDataTypeStr=Inherit: Same as input  ParamDataTypeStr=Inherit: Same as input
  Kp : Gain  Gain=Kp  OutDataTypeStr=Inherit: Same as input  ParamDataTypeStr=Inherit: Same as input
  Logical Operator : Logic  AllPortsSameDT=off  OutDataTypeStr=boolean
  Product : Product  RndMeth=Zero
  Saturation2 : Saturate  UpperLimit=UpperLimit  LowerLimit=LowerLimit
  Sum : Sum  Inputs=|+-  OutDataTypeStr=Inherit: Same as first input
  Sum1 : Sum  Inputs=+-  OutDataTypeStr=Inherit: Same as first input
  Sum6 : Sum  InputSameDT=on  SaturateOnIntegerOverflow=on  OutDataTypeStr=Inherit: Same as first input
  Switch : Switch  Criteria=u2 > Threshold
  Out : Outport
  wires:
  Compare To Zero/1 -> Logical Operator/2
  Product/1 -> Compare To Zero/1
  Kc/1 -> Sum/2
  Ki/1 -> Integrator/1
  Saturation2/1 -> Out/1, Sum1/2
  Kp/1 -> Sum6/1
  Sum6/1 -> Product/2, Sum1/1, Saturation2/1
  Integrator/1 -> Sum6/2, Display/1
  Sum1/1 -> Kc/1, Logical Operator/1
  Error/1 -> Kp/1, Product/1, Sum/1, Switch/3
  Logical Operator/1 -> Switch/2
  Sum/1 -> Switch/1
  Switch/1 -> Ki/1

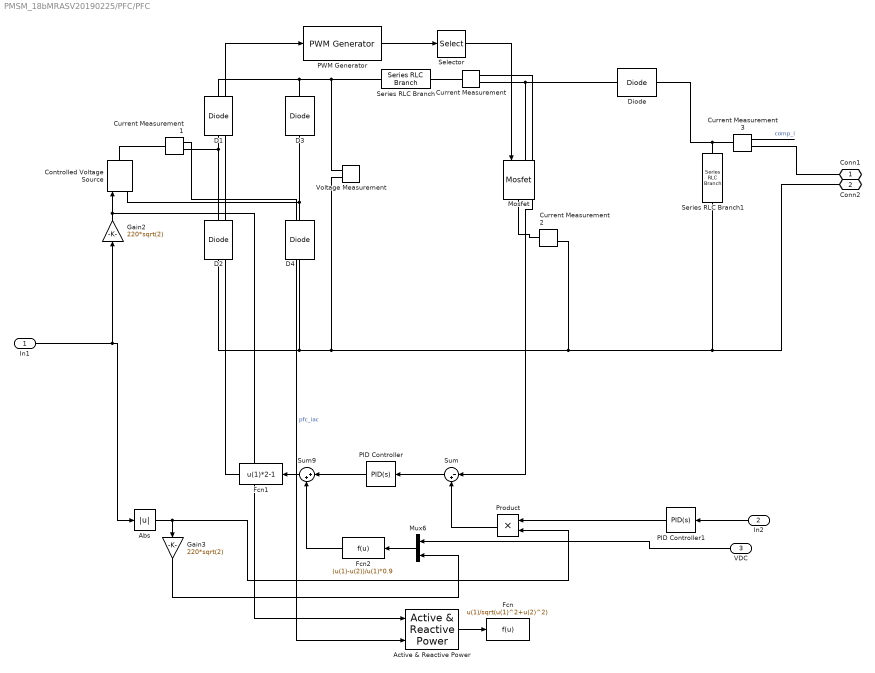
== system PMSM_18bMRASV20190225/PFC/PFC ==
  In1 : Inport
  In2 : Inport  Port=2
  VDC : Inport  Port=3
  Abs : Abs
  Active & Reactive Power : powerlib_extras/Measurements/Active & Reactive Power  f1=50
      settings: SourceProductBaseCode=PS
  Controlled Voltage Source : powerlib/Electrical Sources/Controlled Voltage Source  Initialize=on  Source_Type=AC  Amplitude=0  Phase=0  Frequency=0  Measurements=None
  Current Measurement{,1..3} (4 alike) : powerlib/Measurements/Current Measurement  PhasorSimulation=off  OutputType=Complex  PSBequivalent=0
  D{1..4} (4 alike) : powerlib/Power Electronics/Diode  Ron=0.001  Lon=0  Vf=0.8  IC=0  UseSnubber=off  Rs=500  Cs=250e-9  Measurements=off
  Diode : powerlib/Power Electronics/Diode  Ron=0.001  Lon=0  Vf=0.8  IC=0  UseSnubber=off  Rs=500  Cs=250e-9  Measurements=off
  Fcn : Fcn  Expr=u(1)/sqrt(u(1)^2+u(2)^2)
  Fcn1 : Fcn  Expr=u(1)*2-1
  Fcn2 : Fcn  Expr=(u(1)-u(2))/u(1)*0.9
  Gain2 : Gain  Gain=220*sqrt(2)
  Gain3 : Gain  Gain=220*sqrt(2)
  Mosfet : powerlib/Power Electronics/Mosfet  Ron=0.1  Lon=0  Rd=0.01  Vfd=0  IC=0  Rs=1e5  Cs=inf  Measurements=off
  Mux6 : Mux  Inputs=2
  PID Controller : simulink/Continuous/PID Controller  Controller=PID  Form=Parallel  TimeDomain=Continuous-time  UseExternalTs=off  SampleTime=1  IntegratorMethod=Forward Euler  FilterMethod=Forward Euler  ControllerParametersSource=internal  P=0.2  I=10  D=0  UseFilter=on  N=100  TunerSelectOption=Transfer Function Based (PID Tuner App)  InitialConditionSource=internal  InitialConditionForIntegrator=0  InitialConditionForFilter=0  DifferentiatorICPrevScaledInput=0  ExternalReset=none  TrackingMode=off  Kt=1  LimitOutput=on  UpperSaturationLimit=1  LowerSaturationLimit=-1  LinearizeAsGain=off  AntiWindupMode=none  Kb=1  POutMin=[]  POutMax=[]  IOutMin=[]  IOutMax=[]  DOutMin=[]  DOutMax=[]  NOutMin=[]  NOutMax=[]  SumOutMin=[]  SumOutMax=[]  SaturationOutMin=[]  SaturationOutMax=[]  PParamMin=[]  PParamMax=[]  IParamMin=[]  IParamMax=[]  DParamMin=[]  DParamMax=[]  NParamMin=[]  NParamMax=[]  KbParamMin=[]  KbParamMax=[]  KtParamMin=[]  KtParamMax=[]  KbOutMin=[]  KbOutMax=[]  KtOutMin=[]  KtOutMax=[]  IntegratorOutMin=[]  IntegratorOutMax=[]  FilterOutMin=[]  FilterOutMax=[]  SumI1OutMin=[]  SumI1OutMax=[]  SumI2OutMin=[]  SumI2OutMax=[]  SumI3OutMin=[]  SumI3OutMax=[]  SumI4OutMin=[]  SumI4OutMax=[]  SumDOutMin=[]  SumDOutMax=[]  DifferentiatorOutMin=[]  DifferentiatorOutMax=[]  FilterDiffOutCoefMin=[]  FilterDiffOutCoefMax=[]  ReciprocalOutMin=[]  ReciprocalOutMax=[]  SumDenOutMin=[]  SumDenOutMax=[]  SumNumOutMin=[]  SumNumOutMax=[]  DivideOutMin=[]  DivideOutMax=[]  UdiffTsProdOutMin=[]  UdiffTsProdOutMax=[]  NTsProdOutMin=[]  NTsProdOutMax=[]  UintegralTsProdOutMin=[]  UintegralTsProdOutMax=[]  UngainTsProdOutMin=[]  UngainTsProdOutMax=[]  IntegratorContinuousStateAttributes=''  IntegratorStateMustResolveToSignalObject=off  IntegratorRTWStateStorageClass=Auto  FilterContinuousStateAttributes=''  FilterStateMustResolveToSignalObject=off  FilterRTWStateStorageClass=Auto  ParallelPVariant=InternalParameters  IdealPVariant=Disabled  IVariant=InternalParameters  DVariant=InternalParameters  IntegratorVariant=Continuous  SatVariant=Enabled  AWVariant=Passthrough  PCopyVariant=Disabled  TRVariant=Disabled  FdbkBlocksVariant=Forward  IdealPFdbkVariant=Disabled  SatFdbkVariant=Disabled  DerivativeFilterVariant=ContFilter  NVariant=InternalParameters  NCopyVariant=Disabled  FilterICVariant=InternalICsFilter  IntegratorICVariant=InternalICs  ExternalResetVariant=Disabled  TRSumVariant=Passthrough  SumFdbkVariant=Disabled  SumVariant=Sum_PID  TsampFilterVariant=InternalTs  TsampNgainVariant=Passthrough  TsampIntegralVariant=Passthrough
  PID Controller1 : simulink/Continuous/PID Controller  Controller=PID  Form=Parallel  TimeDomain=Continuous-time  UseExternalTs=off  SampleTime=1  IntegratorMethod=Forward Euler  FilterMethod=Forward Euler  ControllerParametersSource=internal  P=0.25  I=2  D=0  UseFilter=on  N=100  TunerSelectOption=Transfer Function Based (PID Tuner App)  InitialConditionSource=internal  InitialConditionForIntegrator=0  InitialConditionForFilter=0  DifferentiatorICPrevScaledInput=0  ExternalReset=none  TrackingMode=off  Kt=1  LimitOutput=on  UpperSaturationLimit=20  LowerSaturationLimit=0  LinearizeAsGain=off  AntiWindupMode=none  Kb=1  POutMin=[]  POutMax=[]  IOutMin=[]  IOutMax=[]  DOutMin=[]  DOutMax=[]  NOutMin=[]  NOutMax=[]  SumOutMin=[]  SumOutMax=[]  SaturationOutMin=[]  SaturationOutMax=[]  PParamMin=[]  PParamMax=[]  IParamMin=[]  IParamMax=[]  DParamMin=[]  DParamMax=[]  NParamMin=[]  NParamMax=[]  KbParamMin=[]  KbParamMax=[]  KtParamMin=[]  KtParamMax=[]  KbOutMin=[]  KbOutMax=[]  KtOutMin=[]  KtOutMax=[]  IntegratorOutMin=[]  IntegratorOutMax=[]  FilterOutMin=[]  FilterOutMax=[]  SumI1OutMin=[]  SumI1OutMax=[]  SumI2OutMin=[]  SumI2OutMax=[]  SumI3OutMin=[]  SumI3OutMax=[]  SumI4OutMin=[]  SumI4OutMax=[]  SumDOutMin=[]  SumDOutMax=[]  DifferentiatorOutMin=[]  DifferentiatorOutMax=[]  FilterDiffOutCoefMin=[]  FilterDiffOutCoefMax=[]  ReciprocalOutMin=[]  ReciprocalOutMax=[]  SumDenOutMin=[]  SumDenOutMax=[]  SumNumOutMin=[]  SumNumOutMax=[]  DivideOutMin=[]  DivideOutMax=[]  UdiffTsProdOutMin=[]  UdiffTsProdOutMax=[]  NTsProdOutMin=[]  NTsProdOutMax=[]  UintegralTsProdOutMin=[]  UintegralTsProdOutMax=[]  UngainTsProdOutMin=[]  UngainTsProdOutMax=[]  IntegratorContinuousStateAttributes=''  IntegratorStateMustResolveToSignalObject=off  IntegratorRTWStateStorageClass=Auto  FilterContinuousStateAttributes=''  FilterStateMustResolveToSignalObject=off  FilterRTWStateStorageClass=Auto  ParallelPVariant=InternalParameters  IdealPVariant=Disabled  IVariant=InternalParameters  DVariant=InternalParameters  IntegratorVariant=Continuous  SatVariant=Enabled  AWVariant=Passthrough  PCopyVariant=Disabled  TRVariant=Disabled  FdbkBlocksVariant=Forward  IdealPFdbkVariant=Disabled  SatFdbkVariant=Disabled  DerivativeFilterVariant=ContFilter  NVariant=InternalParameters  NCopyVariant=Disabled  FilterICVariant=InternalICsFilter  IntegratorICVariant=InternalICs  ExternalResetVariant=Disabled  TRSumVariant=Passthrough  SumFdbkVariant=Disabled  SumVariant=Sum_PID  TsampFilterVariant=InternalTs  TsampNgainVariant=Passthrough  TsampIntegralVariant=Passthrough
  PWM Generator : powerlib_extras/Control  Blocks/PWM Generator  GeneratorMode="1-arm  bridge (2 pulses)"  Fc=40000  Internal=off  mIndex=0.4  Freq=60  Phase=0
      settings: SourceProductBaseCode=PS
  Product : Product  RndMeth=Zero
  Selector : Selector  InputPortWidth=2  IndexOptions=Index vector (dialog)  Indices=[1]  OutputSizes=1
  Series RLC Branch : powerlib/Elements/Series RLC Branch  LConnTagsString=__new0  RConnTagsString=__new0  BranchType=L  Resistance=1  Inductance=400e-6  SetiL0=off  InitialCurrent=20  Capacitance=1e-6  Setx0=off  InitialVoltage=0  Measurements=None
  Series RLC Branch1 : powerlib/Elements/Series RLC Branch  LConnTagsString=__new0  RConnTagsString=__new0  BranchType=C  Resistance=1  Inductance=5e-3  SetiL0=off  InitialCurrent=20  Capacitance=470e-6*2  Setx0=on  InitialVoltage=300  Measurements=None
  Sum : Sum  Inputs=|-+
  Sum9 : Sum  Inputs=|++
  Voltage Measurement : powerlib/Measurements/Voltage Measurement  PhasorSimulation=off  OutputType=Complex  PSBequivalent=0
  Conn1 : PMIOPort  Side=Right
  Conn2 : PMIOPort  Port=2  Side=Right
  wires:
  Sum9/1 -> Fcn1/1
  Gain2/1 -> Controlled Voltage Source/1, Active & Reactive Power/1
  Current Measurement/1 -> Sum/1
  Gain3/1 -> Mux6/2
  Abs/1 -> Gain3/1, Product/2
  Sum/1 -> PID Controller/1
  PID Controller1/1 -> Product/1
  Fcn1/1 -> PWM Generator/1
  Mux6/1 -> Fcn2/1
  In1/1 -> Abs/1, Gain2/1
  Fcn2/1 -> Sum9/2
  Active & Reactive Power/1 -> Fcn/1
  Current Measurement1/1 -> Active & Reactive Power/2  "pfc_iac"
  PWM Generator/1 -> Selector/1
  Selector/1 -> Mosfet/1
  Product/1 -> Sum/2
  PID Controller/1 -> Sum9/1
  VDC/1 -> Mux6/1
  In2/1 -> PID Controller1/1
  Current Measurement3/1 -> ?  "comp_i"
  connections:
  D3/RConn1 -- Series RLC Branch/LConn1 -- Voltage Measurement/LConn1 -- D1/RConn1
  Voltage Measurement/LConn2 -- D2/LConn1 -- D4/LConn1 -- Conn2/RConn1 -- Series RLC Branch1/RConn1 -- Current Measurement2/RConn1
  Current Measurement/RConn1 -- Diode/LConn1 -- Mosfet/LConn1
  Current Measurement/LConn1 -- Series RLC Branch/RConn1
  Current Measurement2/LConn1 -- Mosfet/RConn1
  Current Measurement1/RConn1 -- D2/RConn1 -- D1/LConn1
  Series RLC Branch1/LConn1 -- Current Measurement3/LConn1 -- Diode/RConn1
  Controlled Voltage Source/LConn1 -- D3/LConn1 -- D4/RConn1
  Current Measurement1/LConn1 -- Controlled Voltage Source/RConn1
  Current Measurement3/RConn1 -- Conn1/RConn1

== system PMSM_18bMRASV20190225/SVPWM/SVPWM ==
  Ualfa : Inport
  Ubeta : Inport  Port=2
  VDC : Inport  Port=3
  Frequence : Constant  Value=0.001/F
  N1 : Subsystem
  Subsystem : Subsystem
  Subsystem1 : Subsystem
  X.Y.Z : Subsystem
  produce PWM : Subsystem
  pulse : Outport  VectorParamsAs1DForOutWhenUnconnected=off
  wires:
  Ubeta/1 -> X.Y.Z/3(Ubeta), N1/2(Ubeta)
  Subsystem/2(T2) -> Subsystem1/2(T2)
  Subsystem/1(T1) -> Subsystem1/1(T1)
  Ualfa/1 -> N1/1(Ualfa), X.Y.Z/2(Ualfa)
  Subsystem1/3(Tcm3) -> produce PWM/3(Tcm3)
  Subsystem1/2(Tcm2) -> produce PWM/2(Tcm2)
  Subsystem1/1(Tcm1) -> produce PWM/1(Tcm1)
  X.Y.Z/3(Z) -> Subsystem/4(Z)
  X.Y.Z/2(Y) -> Subsystem/3(Y)
  X.Y.Z/1(X) -> Subsystem/2(X)
  N1/1(N) -> Subsystem1/4(N), Subsystem/1(N)
  VDC/1 -> X.Y.Z/4(Udc)
  Frequence/1 -> Subsystem/5(T), Subsystem1/3(T), X.Y.Z/1(T)
  produce PWM/1(pulse) -> pulse/1

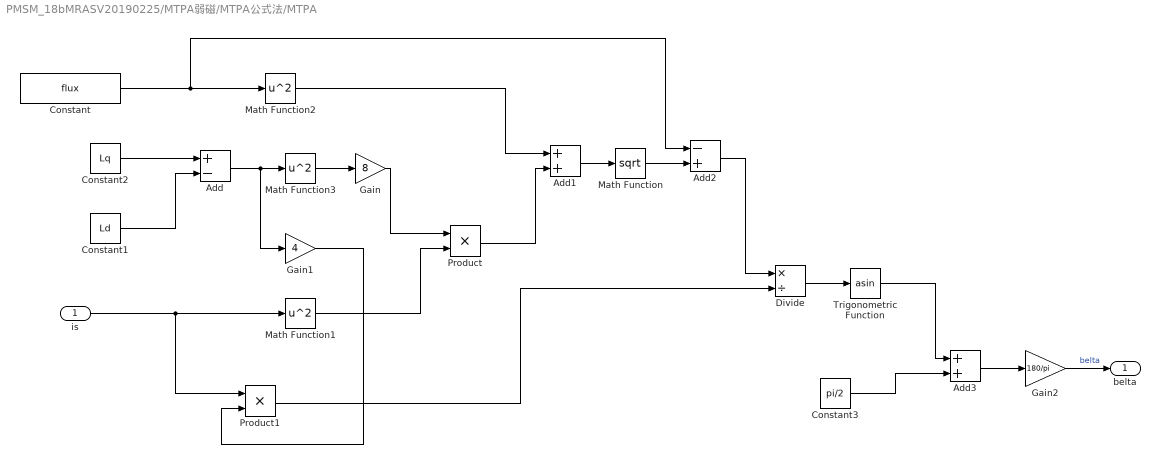
== system PMSM_18bMRASV20190225/MTPA弱磁/MTPA公式法/MTPA ==
  is : Inport
  Add : Sum  Inputs=+-
  Add1 : Sum
  Add2 : Sum  Inputs=-+
  Add3 : Sum
  Constant : Constant  Value=flux
  Constant1 : Constant  Value=Ld
  Constant2 : Constant  Value=Lq
  Constant3 : Constant  Value=pi/2
  Divide : Product  Inputs=*/
  Gain : Gain  Gain=8
  Gain1 : Gain  Gain=4
  Gain2 : Gain  Gain=180/pi
  Math Function : Math  Operator=sqrt  SignedPower=on  SaturateOnIntegerOverflow=on
  Math Function1 : Math  Operator=square  SignedPower=on  SaturateOnIntegerOverflow=on
  Math Function2 : Math  Operator=square  SignedPower=on  SaturateOnIntegerOverflow=on
  Math Function3 : Math  Operator=square  SignedPower=on  SaturateOnIntegerOverflow=on
  Product : Product  RndMeth=Zero
  Product1 : Product  RndMeth=Zero
  Trigonometric Function : Trigonometry  Operator=asin
  belta : Outport
  wires:
  Add3/1 -> Gain2/1
  Constant3/1 -> Add3/2
  Trigonometric Function/1 -> Add3/1
  Divide/1 -> Trigonometric Function/1
  Product1/1 -> Divide/2
  Gain1/1 -> Product1/2
  Add2/1 -> Divide/1
  Add1/1 -> Math Function/1
  Product/1 -> Add1/2
  Math Function2/1 -> Add1/1
  Math Function1/1 -> Product/2
  Gain/1 -> Product/1
  Math Function3/1 -> Gain/1
  Add/1 -> Math Function3/1, Gain1/1
  is/1 -> Math Function1/1, Product1/1
  Constant/1 -> Math Function2/1, Add2/1
  Constant1/1 -> Add/2
  Constant2/1 -> Add/1
  Gain2/1 -> belta/1  "belta"
  Math Function/1 -> Add2/2

== system PMSM_18bMRASV20190225/MTPA弱磁/MTPA公式法/Subsystem1 ==
  "belta " : Inport
  is : Inport  Port=2
  Gain1 : Gain  Gain=pi/180
  Product : Product  RndMeth=Zero
  Product1 : Product  RndMeth=Zero
  Trigonometric Function : Trigonometry
  Trigonometric Function1 : Trigonometry  Operator=cos
  id : Outport
  iq : Outport  Port=2
  wires:
  Product/1 -> iq/1
  Product1/1 -> id/1
  Trigonometric Function/1 -> Product/1
  Trigonometric Function1/1 -> Product1/1
  "belta "/1 -> Gain1/1
  is/1 -> Product/2, Product1/2
  Gain1/1 -> Trigonometric Function/1, Trigonometric Function1/1

== system PMSM_18bMRASV20190225/SVPWM/SVPWM/N1 ==
  Ualfa : Inport
  Ubeta : Inport  Port=2
  Constant : Constant
  Constant1 : Constant  Value=0
  Gain : Gain  Gain=1.732
  Gain1 : Gain  Gain=-1.732
  Gain2 : Gain  Gain=2
  Gain3 : Gain  Gain=4
  Sum : Sum  Inputs=|-+
  Sum1 : Sum  Inputs=|-+
  Sum2 : Sum  Inputs=|+++
  Switch : Switch
  Switch1 : Switch
  Switch2 : Switch
  N : Outport  VectorParamsAs1DForOutWhenUnconnected=off
  wires:
  Sum2/1 -> N/1
  Gain3/1 -> Sum2/3
  Switch/1 -> Sum2/1
  Gain2/1 -> Sum2/2
  Switch2/1 -> Gain3/1
  Switch1/1 -> Gain2/1
  Constant1/1 -> Switch2/3, Switch1/3, Switch/3
  Gain1/1 -> Sum1/2
  Sum1/1 -> Switch2/2
  Sum/1 -> Switch1/2
  Gain/1 -> Sum/2
  Ualfa/1 -> Gain/1, Gain1/1
  Constant/1 -> Switch1/1, Switch2/1, Switch/1
  Ubeta/1 -> Sum1/1, Sum/1, Switch/2

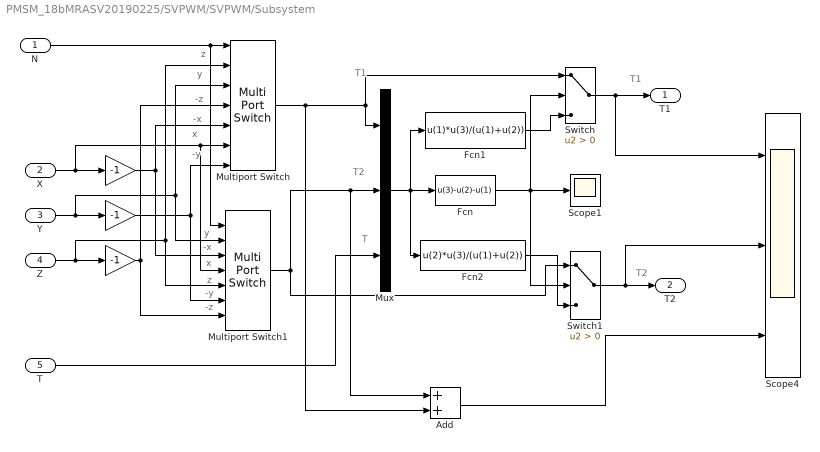
== system PMSM_18bMRASV20190225/SVPWM/SVPWM/Subsystem ==
  note: T2
  note: T1
  note: T
  note: T2
  note: T1
  note: -z
  note: -y
  note: z
  note: x
  note: -x
  note: y
  note: -y
  note: x
  note: -x
  note: -z
  note: y
  note: z
  N : Inport
  X : Inport  Port=2
  Y : Inport  Port=3
  Z : Inport  Port=4
  T : Inport  Port=5
  " " : Gain  Gain=-1
  "  " : Gain  Gain=-1
  "    " : Gain  Gain=-1
  Add : Sum
  Fcn : Fcn  Expr=u(3)-u(2)-u(1)
  Fcn1 : Fcn  Expr=u(1)*u(3)/(u(1)+u(2))
  Fcn2 : Fcn  Expr=u(2)*u(3)/(u(1)+u(2))
  Multiport Switch : MultiPortSwitch  Inputs=6  DiagnosticForDefault=None
  Multiport Switch1 : MultiPortSwitch  Inputs=6  DiagnosticForDefault=None
  Mux : Mux  Inputs=3
  Scope1 : Scope
  Scope4 : Scope  NumInputPorts=3
  Switch : Switch  Criteria=u2 > Threshold
  Switch1 : Switch  Criteria=u2 > Threshold
  T1 : Outport  VectorParamsAs1DForOutWhenUnconnected=off
  T2 : Outport  Port=2  VectorParamsAs1DForOutWhenUnconnected=off
  wires:
  Add/1 -> Scope4/3
  Switch1/1 -> Scope4/2, T2/1
  Switch/1 -> Scope4/1, T1/1
  Fcn2/1 -> Switch1/3
  Fcn1/1 -> Switch/3
  Mux/1 -> Fcn2/1, Fcn1/1, Fcn/1
  T/1 -> Mux/3
  Multiport Switch/1 -> Add/2, Switch/1, Mux/1
  " "/1 -> Multiport Switch1/3, Multiport Switch/5
  "  "/1 -> Multiport Switch1/6, Multiport Switch/7
  "    "/1 -> Multiport Switch/4, Multiport Switch1/7
  Z/1 -> "    "/1, Multiport Switch/2, Multiport Switch1/5
  Y/1 -> "  "/1, Multiport Switch/3, Multiport Switch1/2
  X/1 -> " "/1, Multiport Switch/6, Multiport Switch1/4
  N/1 -> Multiport Switch/1, Multiport Switch1/1
  Fcn/1 -> Scope1/1, Switch1/2, Switch/2
  Multiport Switch1/1 -> Add/1, Mux/2, Switch1/1

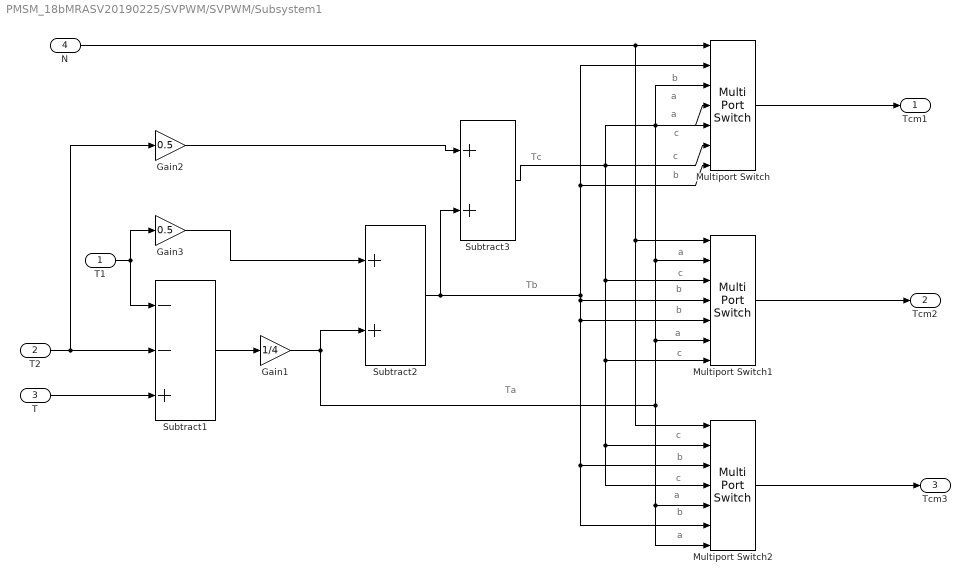
== system PMSM_18bMRASV20190225/SVPWM/SVPWM/Subsystem1 ==
  note: a
  note: b
  note: a
  note: c
  note: b
  note: c
  note: c
  note: a
  note: b
  note: b
  note: c
  note: a
  note: b
  note: c
  note: c
  note: a
  note: a
  note: b
  note: Tc
  note: Tb
  note: Ta
  T1 : Inport
  T2 : Inport  Port=2
  T : Inport  Port=3
  N : Inport  Port=4
  Gain1 : Gain  Gain=1/4
  Gain2 : Gain  Gain=0.5
  Gain3 : Gain  Gain=0.5
  Multiport Switch : MultiPortSwitch  Inputs=6  DiagnosticForDefault=None
  Multiport Switch1 : MultiPortSwitch  Inputs=6  DiagnosticForDefault=None
  Multiport Switch2 : MultiPortSwitch  Inputs=6  DiagnosticForDefault=None
  Subtract1 : Sum  Inputs=--+
  Subtract2 : Sum
  Subtract3 : Sum
  Tcm1 : Outport  VectorParamsAs1DForOutWhenUnconnected=off
  Tcm2 : Outport  Port=2  VectorParamsAs1DForOutWhenUnconnected=off
  Tcm3 : Outport  Port=3  VectorParamsAs1DForOutWhenUnconnected=off
  wires:
  Subtract3/1 -> Multiport Switch2/4, Multiport Switch2/2, Multiport Switch1/7, Multiport Switch1/3, Multiport Switch/6, Multiport Switch/5
  N/1 -> Multiport Switch1/1, Multiport Switch2/1, Multiport Switch/1
  Gain2/1 -> Subtract3/1
  Subtract2/1 -> Multiport Switch2/6, Multiport Switch2/3, Multiport Switch1/5, Multiport Switch1/4, Multiport Switch/7, Multiport Switch/2, Subtract3/2
  Gain1/1 -> Subtract2/2, Multiport Switch1/6, Multiport Switch1/2, Multiport Switch/4, Multiport Switch/3, Multiport Switch2/7, Multiport Switch2/5
  Subtract1/1 -> Gain1/1
  Gain3/1 -> Subtract2/1
  T1/1 -> Subtract1/1, Gain3/1
  T/1 -> Subtract1/3
  T2/1 -> Subtract1/2, Gain2/1
  Multiport Switch/1 -> Tcm1/1
  Multiport Switch1/1 -> Tcm2/1
  Multiport Switch2/1 -> Tcm3/1

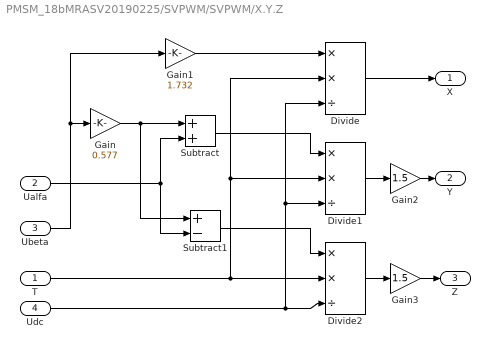
== system PMSM_18bMRASV20190225/SVPWM/SVPWM/X.Y.Z ==
  T : Inport
  Ualfa : Inport  Port=2
  Ubeta : Inport  Port=3
  Udc : Inport  Port=4
  Divide : Product  Inputs=**/
  Divide1 : Product  Inputs=**/
  Divide2 : Product  Inputs=**/
  Gain : Gain  Gain=0.577
  Gain1 : Gain  Gain=1.732
  Gain2 : Gain  Gain=1.5
  Gain3 : Gain  Gain=1.5
  Subtract : Sum
  Subtract1 : Sum  Inputs=+-
  X : Outport  VectorParamsAs1DForOutWhenUnconnected=off
  Y : Outport  Port=2  VectorParamsAs1DForOutWhenUnconnected=off
  Z : Outport  Port=3  VectorParamsAs1DForOutWhenUnconnected=off
  wires:
  Ubeta/1 -> Gain/1, Gain1/1
  Gain3/1 -> Z/1
  Gain2/1 -> Y/1
  Divide2/1 -> Gain3/1
  Divide1/1 -> Gain2/1
  Divide/1 -> X/1
  Subtract1/1 -> Divide2/1
  Subtract/1 -> Divide1/1
  Ualfa/1 -> Subtract/2, Subtract1/2
  Udc/1 -> Divide/3, Divide1/3, Divide2/3
  T/1 -> Divide/2, Divide1/2, Divide2/2
  Gain1/1 -> Divide/1
  Gain/1 -> Subtract1/1, Subtract/1

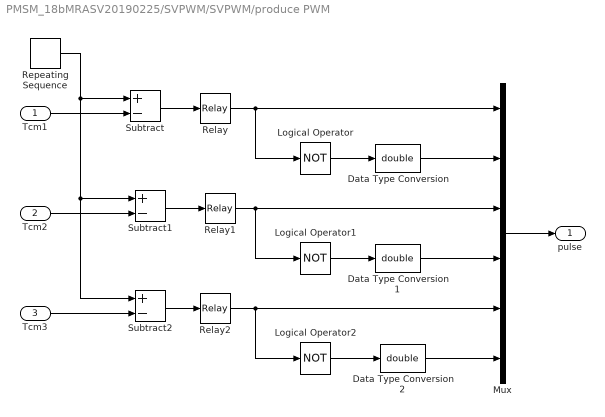
== system PMSM_18bMRASV20190225/SVPWM/SVPWM/produce PWM ==
  Tcm1 : Inport
  Tcm2 : Inport  Port=2
  Tcm3 : Inport  Port=3
  Data Type Conversion : DataTypeConversion  OutDataTypeStr=double
  Data Type Conversion1 : DataTypeConversion  OutDataTypeStr=double
  Data Type Conversion2 : DataTypeConversion  OutDataTypeStr=double
  Logical Operator : Logic  Operator=NOT  AllPortsSameDT=off
  Logical Operator1 : Logic  Operator=NOT  AllPortsSameDT=off
  Logical Operator2 : Logic  Operator=NOT  AllPortsSameDT=off
  Mux : Mux  Inputs=6
  Relay : Relay
  Relay1 : Relay
  Relay2 : Relay
  Repeating Sequence : simulink/Sources/Repeating Sequence  rep_seq_t=[0 0.001/F 0.002/F]  rep_seq_y=[0 0.001/F 0]
  Subtract : Sum  Inputs=+-
  Subtract1 : Sum  Inputs=+-
  Subtract2 : Sum  Inputs=+-
  pulse : Outport  VectorParamsAs1DForOutWhenUnconnected=off
  wires:
  Data Type Conversion2/1 -> Mux/6
  Data Type Conversion1/1 -> Mux/4
  Data Type Conversion/1 -> Mux/2
  Mux/1 -> pulse/1
  Relay2/1 -> Mux/5, Logical Operator2/1
  Relay1/1 -> Mux/3, Logical Operator1/1
  Relay/1 -> Mux/1, Logical Operator/1
  Logical Operator/1 -> Data Type Conversion/1
  Logical Operator2/1 -> Data Type Conversion2/1
  Logical Operator1/1 -> Data Type Conversion1/1
  Tcm3/1 -> Subtract2/2
  Tcm2/1 -> Subtract1/2
  Tcm1/1 -> Subtract/2
  Repeating Sequence/1 -> Subtract1/1, Subtract2/1, Subtract/1
  Subtract2/1 -> Relay2/1
  Subtract1/1 -> Relay1/1
  Subtract/1 -> Relay/1
